simulink model "TestCompareUnit8"  (R2013b)
settings: Solver=ode45  StartTime=0.0  StopTime=10.0  RelTol=1e-3
libraries: simulink x1
settings Model: Creator=Think79  LastModifiedBy=Think79

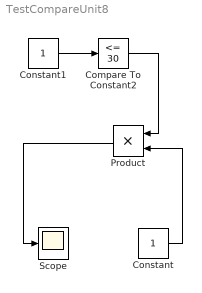
== system TestCompareUnit8 ==
  Compare To Constant2 : simulink/Logic and Bit Operations/Compare To Constant  relop=<=  const=30  OutDataTypeStr=uint8
  Constant : Constant
  Constant1 : Constant
  Product : Product
  Scope : Scope
  wires:
  Compare To Constant2/1 -> Product/1
  Constant/1 -> Product/2
  Constant1/1 -> Compare To Constant2/1
  Product/1 -> Scope/1
